simulink model "parse_in_test"  (R2013b)
settings: Solver=ode45  StartTime=0.0  StopTime=40  RelTol=1e-3
libraries: xbsIndex_r4 x16, xps_library x1
settings Model: Creator=root  LastModifiedBy=root

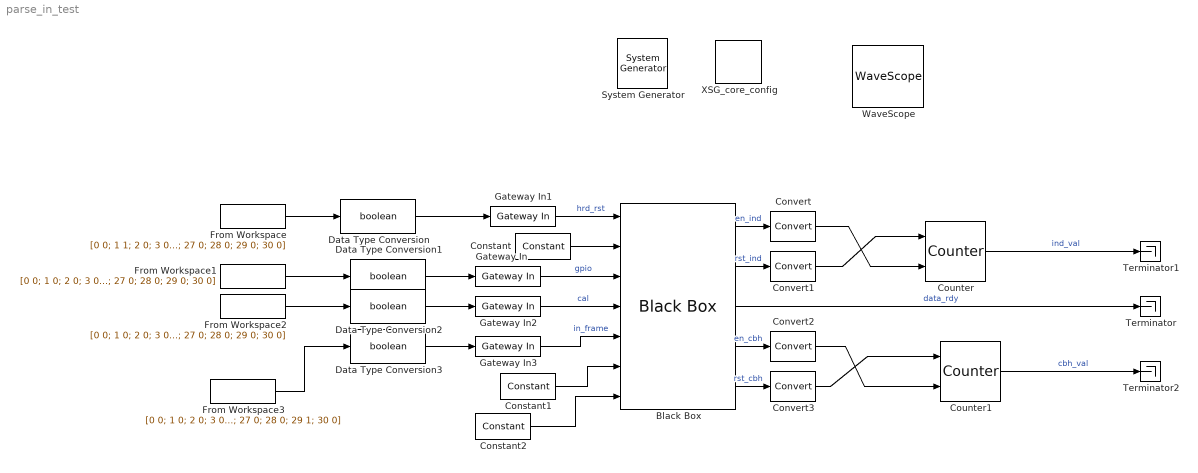
== system parse_in_test ==
  " System Generator" : xbsIndex_r4/ System Generator  Tag=genX  xilinxfamily=Kintex7  part=xc7k325t  speed=-3  package=fbg676  synthesis_tool=XST  clock_wrapper=Clock Enables  directory=./netlist  proj_type=Project Navigator  Synth_file=XST Defaults  Impl_file=ISE Defaults  testbench=off  simulink_period=1  sysclk_period=10  dcm_input_clock_period=10  incr_netlist=off  trim_vbits=Everywhere in SubSystem  dbl_ovrd=According to Block Masks  core_generation=According to Block Masks  run_coregen=off  deprecated_control=off  eval_field=0  block_type=sysgen
  Black Box : xbsIndex_r4/Black Box  init_code=parse_inputs_config  sim_method=ISE Simulator  verbose=off  block_type=blackbox2
  Constant : xbsIndex_r4/Constant  const=0  gui_display_data_type=Boolean  arith_type=Boolean  n_bits=16  bin_pt=14  preci_type=Single  exp_width=8  frac_width=24  explicit_period=on  period=1  equ=P=C  opselect=C  inp2=PCIN>>17  opr=+  inp1=P  carry=CIN  dbl_ovrd=off  block_type=constant
  Constant1 : xbsIndex_r4/Constant  const=0  gui_display_data_type=Boolean  arith_type=Boolean  n_bits=16  bin_pt=14  preci_type=Single  exp_width=8  frac_width=24  explicit_period=on  period=1  equ=P=C  opselect=C  inp2=PCIN>>17  opr=+  inp1=P  carry=CIN  dbl_ovrd=off  block_type=constant
  Constant2 : xbsIndex_r4/Constant  const=0  gui_display_data_type=Boolean  arith_type=Boolean  n_bits=16  bin_pt=14  preci_type=Single  exp_width=8  frac_width=24  explicit_period=on  period=1  equ=P=C  opselect=C  inp2=PCIN>>17  opr=+  inp1=P  carry=CIN  dbl_ovrd=off  block_type=constant
  Convert{,1..3} (4 alike) : xbsIndex_r4/Convert  gui_display_data_type=Boolean  arith_type=Boolean  n_bits=16  bin_pt=14  float_type=Single  exp_bits=8  fraction_bits=24  quantization=Truncate  overflow=Wrap  en=off  latency=0  dbl_ovrd=off  pipeline=off  block_type=convert
  Counter : xbsIndex_r4/Counter  cnt_type=Free Running  cnt_to=Inf  operation=Up  start_count=0  cnt_by_val=1  arith_type=Unsigned  n_bits=8  bin_pt=0  load_pin=off  rst=on  en=on  explicit_period=on  period=1  dbl_ovrd=off  use_behavioral_HDL=off  implementation=Fabric  block_type=counter
  Counter1 : xbsIndex_r4/Counter  cnt_type=Free Running  cnt_to=Inf  operation=Up  start_count=0  cnt_by_val=1  arith_type=Unsigned  n_bits=8  bin_pt=0  load_pin=off  rst=on  en=on  explicit_period=on  period=1  dbl_ovrd=off  use_behavioral_HDL=off  implementation=Fabric  block_type=counter
  Data Type Conversion{,1..3} (4 alike) : DataTypeConversion  OutDataTypeStr=boolean
  From Workspace : FromWorkspace  VariableName=[0 0; 1 1; 2 0; 3 0; 4 0; 5 0; 6 0; 7 0; 8 0; 9 0; 10 0; 11 0; 12 0; 13 0; 14 0; 15 0; 16 0; 17 0; 18 0; 19 0; 20 0; 21 0; 22 0; 23 0; 24 0; 25 0; 26 0; 27 0; 28 0; 29 0; 30 0]  OutDataTypeStr=double  SampleTime=1
  From Workspace1 : FromWorkspace  VariableName=[0 0; 1 0; 2 0; 3 0; 4 0; 5 0; 6 0; 7 0; 8 0; 9 1; 10 1; 11 1; 12 1; 13 1; 14 1; 15 0; 16 0; 17 0; 18 0; 19 0; 20 0; 21 0; 22 0; 23 0; 24 1; 25 1; 26 1; 27 0; 28 0; 29 0; 30 0]  OutDataTypeStr=double  SampleTime=1  OutputAfterFinalValue=Holding final value
  From Workspace2 : FromWorkspace  VariableName=[0 0; 1 0; 2 0; 3 0; 4 0; 5 0; 6 1; 7 0; 8 0; 9 0; 10 0; 11 0; 12 0; 13 0; 14 0; 15 0; 16 0; 17 0; 18 0; 19 0; 20 0; 21 0; 22 0; 23 0; 24 0; 25 0; 26 0; 27 0; 28 0; 29 0; 30 0]  OutDataTypeStr=double  SampleTime=1
  From Workspace3 : FromWorkspace  VariableName=[0 0; 1 0; 2 0; 3 0; 4 0; 5 0; 6 0; 7 0; 8 0; 9 0; 10 0; 11 0; 12 0; 13 0; 14 0; 15 0; 16 0; 17 0; 18 1; 19 0; 20 0; 21 0; 22 0; 23 0; 24 0; 25 0; 26 0; 27 0; 28 0; 29 1; 30 0]  OutDataTypeStr=double  SampleTime=1  OutputAfterFinalValue=Holding final value
  Gateway In{,1..3} (4 alike) : xbsIndex_r4/Gateway In  gui_display_data_type=Boolean  arith_type=Boolean  n_bits=16  bin_pt=14  preci_type=Single  exp_width=8  frac_width=24  quantization="Round  (unbiased: +/- Inf)"  overflow=Saturate  period=1  dbl_ovrd=off  timing_constraint=None  locs_specified=off  LOCs={}  UseAsADC=off  ADCChannel='1'  inherit_from_input=off  hdl_port=on  block_type=gatewayin
  Terminator : Terminator
  Terminator1 : Terminator
  Terminator2 : Terminator
  WaveScope : xbsIndex_r4/WaveScope  block_type=wavescope
  XSG_core_config : xps_library/XSG_core_config  Tag=xps:xsg  hw_sys=ROACH2:sx475t  clk_src=sys_clk  ROACH_clk_src=sys_clk  ROACH2_clk_src=sys_clk  MKDIG_clk_src=sys_clk  clk_rate=100  sample_period=1  synthesis_tool=XST
  wires:
  Black Box/1 -> Convert/1  "en_ind"
  Black Box/2 -> Convert1/1  "rst_ind"
  Black Box/4 -> Convert2/1  "en_cbh"
  Black Box/5 -> Convert3/1  "rst_cbh"
  Black Box/3 -> Terminator/1  "data_rdy"
  Counter/1 -> Terminator1/1  "ind_val"
  Counter1/1 -> Terminator2/1  "cbh_val"
  Constant/1 -> Black Box/2
  Constant1/1 -> Black Box/6
  Constant2/1 -> Black Box/7
  Gateway In/1 -> Black Box/3  "gpio"
  Gateway In1/1 -> Black Box/1  "hrd_rst"
  Gateway In2/1 -> Black Box/4  "cal"
  Gateway In3/1 -> Black Box/5  "in_frame"
  From Workspace/1 -> Data Type Conversion/1
  From Workspace1/1 -> Data Type Conversion1/1
  From Workspace2/1 -> Data Type Conversion2/1
  From Workspace3/1 -> Data Type Conversion3/1
  Data Type Conversion/1 -> Gateway In1/1
  Data Type Conversion1/1 -> Gateway In/1
  Data Type Conversion2/1 -> Gateway In2/1
  Data Type Conversion3/1 -> Gateway In3/1
  Convert/1 -> Counter/2
  Convert1/1 -> Counter/1
  Convert2/1 -> Counter1/2
  Convert3/1 -> Counter1/1
